simulink model "O_CloseLoop_Dynmodel"  (R2016b)
settings: Solver=VariableStepAuto  StartTime=0.0  StopTime=60.0  RelTol=1e-3
values from neighbouring files (symbols this model uses):
  MWS = JT9D_setup_everything_Dyn()    [BP_change_deter_data.m]    (also in JT9D_setup_everything_Dyn.m = input_set_0_0_100(MWS); make_train_data.m; sim_all_loss.m)
undefined symbols (not defined in the file or in its folder): Compressor, Lib_Turbo_Compressor_TMATS, stripchar_TMATS
libraries: Lib_Turbo_Duct_TMATS x5, Lib_Solve_DataOut_TMATS x5, Lib_Solve_OuterLoopIntegrator_TMATS x2, Lib_Turbo_Nozzle_TMATS x2, Lib_Turbo_Shaft_TMATS x2, Lib_Cntrl_FirstOrderActuator_TMATS x1, simulink x1, Lib_Cntrl_SimplePIcontroller_TMATS x1, Lib_Solve_IterNRSolverJC_TMATS x1, Lib_Turbo_Ambient_TMATS x1, Lib_Turbo_Burner_TMATS x1, Lib_Turbo_StaticCalc_TMATS x1
(part 1 of 2)
settings Model: Creator=zhang  LastModifiedBy=zhangshu
settings SolverCC: ZeroCrossAlgorithm=Adaptive

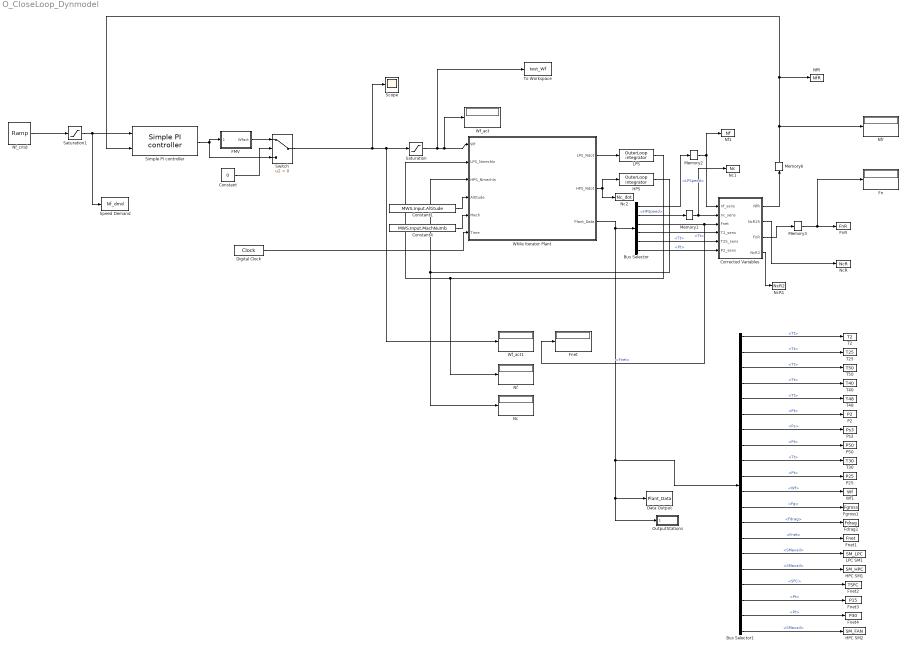
== system O_CloseLoop_Dynmodel ==
  Bus Selector : BusSelector  OutputSignals=Speed.LPSpeed,Speed.HPSpeed,Thrust.Fnet,StationData.S2.Tt,StationData.S24.Tt,StationData.S2.Pt
  Bus Selector1 : BusSelector  OutputSignals=StationData.S2.Tt,StationData.S24.Tt,StationData.S5.Tt,StationData.S4.Tt,StationData.S48.Tt,StationData.S2.Pt,StationData.S3.Ps,StationData.S5.Pt,StationData.S3.Tt,StationData.S24.Pt,Wf,Thrust.Fg,Data.Amb.Fdrag,Thrust.Fnet,Data.LPC.SMavail,Data.HPC.SMavail,SFC,StationData.S17.Pt,StationData.S3.Pt,Data.Fan.SMavail
  Constant : Constant  Value=0
  Constant1 : Constant  Value=MWS.Input.Altitude
  Constant4 : Constant  Value=MWS.Input.MachNumb
  Corrected Variables : Subsystem
  Data Output : ToWorkspace  VariableName=Plant_Data  SaveFormat=Timeseries  SampleTime=-1
  Digital Clock : DigitalClock  SampleTime=0.01
  FMV : Subsystem
  Fdrag1 : ToWorkspace  VariableName=Fdrag  SampleTime=-1
  Fgross1 : ToWorkspace  VariableName=Fgross  SampleTime=-1
  Fn : Display
  FnR : ToWorkspace  VariableName=FnR  SampleTime=-1
  Fnet : Display
  Fnet1 : ToWorkspace  VariableName=Fnet  SampleTime=-1
  Fnet2 : ToWorkspace  VariableName=TSFC  SampleTime=-1
  Fnet3 : ToWorkspace  VariableName=P15  SampleTime=-1
  Fnet4 : ToWorkspace  VariableName=P30  SampleTime=-1
  HPC SM1 : ToWorkspace  VariableName=SM_HPC  SampleTime=-1
  HPC SM2 : ToWorkspace  VariableName=SM_FAN  SampleTime=-1
  HPS : Lib_Solve_OuterLoopIntegrator_TMATS/OuterLoop integrator  OL_IC_M=MWS.Input.HP_Shaft
  LPC SM1 : ToWorkspace  VariableName=SM_LPC  SampleTime=-1
  LPS : Lib_Solve_OuterLoopIntegrator_TMATS/OuterLoop integrator  OL_IC_M=MWS.Input.LP_Shaft
  Memory{1..3,6} (4 alike) : Memory
  Nc : Display
  Nc1 : ToWorkspace  VariableName=Nc  SampleTime=-1
  Nc2 : ToWorkspace  VariableName=Nc_dot  SampleTime=-1
  NcR : ToWorkspace  VariableName=NcR  SampleTime=-1
  NcR1 : ToWorkspace  VariableName=NcR2  SampleTime=-1
  Nf : Display
  Nf1 : ToWorkspace  VariableName=Nf  SampleTime=-1
  NfR : ToWorkspace  VariableName=NfR  SampleTime=-1
  Nf_cmd : simulink/Sources/Ramp  slope=0  start=5  X0=3656.1
  Nfr : Display
  OutputStations : Subsystem
  P2 : ToWorkspace  VariableName=P2  SampleTime=-1
  P25 : ToWorkspace  VariableName=P25  SampleTime=-1
  P50 : ToWorkspace  VariableName=P50  SampleTime=-1
  Ps3 : ToWorkspace  VariableName=Ps3  SampleTime=-1
  Saturation : Saturate  UpperLimit=6  LowerLimit=0.2
  Saturation1 : Saturate  UpperLimit=3800  LowerLimit=1900
  Scope : Scope
  Simple PI controller : Lib_Cntrl_SimplePIcontroller_TMATS/Simple PI controller  Kp_M=0.0011  Ki_M=0.0556  PI_IC_M=MWS.Input.Wfin
  Speed Demand : ToWorkspace  VariableName=Nf_dmd  SaveFormat=Timeseries  SampleTime=-1
  Switch : Switch  Criteria=u2 > Threshold
  T2 : ToWorkspace  VariableName=T2  SampleTime=-1
  T25 : ToWorkspace  VariableName=T25  SampleTime=-1
  T30 : ToWorkspace  VariableName=T30  SampleTime=-1
  T40 : ToWorkspace  VariableName=T40  SampleTime=-1
  T48 : ToWorkspace  VariableName=T48  SampleTime=-1
  T50 : ToWorkspace  VariableName=T50  SampleTime=-1
  To Workspace : ToWorkspace  VariableName=test_Wf  SaveFormat=Timeseries  SampleTime=-1
  Wf1 : ToWorkspace  VariableName=Wf  SampleTime=-1
  Wf_act : Display
  Wf_act1 : Display
  While Iterator Plant : Subsystem  TreatAsAtomicUnit=on
  wires:
  Bus Selector/3 -> Fnet/1, Corrected Variables/3(Fnet)  "<Fnet>"
  Bus Selector/5 -> Corrected Variables/5(T25_sens)  "<Tt>"
  Bus Selector/6 -> Corrected Variables/6(P2_sens)  "<Pt>"
  While Iterator Plant/1(LPS_Ndot) -> LPS/1
  While Iterator Plant/2(HPS_Ndot) -> Nc2/1, HPS/1
  Constant4/1 -> While Iterator Plant/5(Mach)
  Constant1/1 -> While Iterator Plant/4(Altitude)
  Bus Selector1/11 -> Wf1/1  "<Wf>"
  Bus Selector1/3 -> T50/1  "<Tt>"
  Bus Selector1/2 -> T25/1  "<Tt>"
  Bus Selector1/1 -> T2/1  "<Tt>"
  Bus Selector1/4 -> T40/1  "<Tt>"
  Bus Selector1/5 -> T48/1  "<Tt>"
  Bus Selector1/6 -> P2/1  "<Pt>"
  Bus Selector1/7 -> Ps3/1  "<Ps>"
  Bus Selector1/8 -> P50/1  "<Pt>"
  Bus Selector1/9 -> T30/1  "<Tt>"
  Bus Selector1/10 -> P25/1  "<Pt>"
  Bus Selector1/15 -> LPC SM1/1  "<SMavail>"
  Bus Selector1/16 -> HPC SM1/1  "<SMavail>"
  HPS/1 -> Nc/1, While Iterator Plant/3(HPS_NmechIn)
  Corrected Variables/3(FnR) -> Memory3/1
  Memory1/1 -> Nc1/1, Corrected Variables/2(nc_sens)
  Memory2/1 -> Nf1/1, Corrected Variables/1(nf_sens)
  Corrected Variables/2(NcR25) -> NcR/1
  LPS/1 -> Nf/1, While Iterator Plant/2(LPS_NmechIn)
  Memory3/1 -> Fn/1, FnR/1
  Bus Selector/4 -> Corrected Variables/4(T2_sens)  "<Tt>"
  Bus Selector1/12 -> Fgross1/1  "<Fg>"
  Bus Selector1/14 -> Fnet1/1  "<Fnet>"
  Bus Selector1/13 -> Fdrag1/1  "<Fdrag>"
  Switch/1 -> Scope/1, Saturation/1, Wf_act1/1
  Bus Selector/1 -> Memory2/1  "<LPSpeed>"
  Bus Selector/2 -> Memory1/1  "<HPSpeed>"
  While Iterator Plant/3(Plant_Data) -> OutputStations/1(DataBus), Data Output/1, Bus Selector1/1, Bus Selector/1
  Saturation/1 -> To Workspace/1, While Iterator Plant/1(Wf), Wf_act/1
  Bus Selector1/17 -> Fnet2/1  "<SFC>"
  Digital Clock/1 -> While Iterator Plant/6(Time)
  Corrected Variables/1(NfR) -> Memory6/1
  Simple PI controller/1 -> FMV/1(Wfdmd), Switch/3
  FMV/1(Wfact) -> Switch/1
  Constant/1 -> Switch/2
  Memory6/1 -> Simple PI controller/2, NfR/1, Nfr/1
  Nf_cmd/1 -> Saturation1/1
  Corrected Variables/4(NcR2) -> NcR1/1
  Saturation1/1 -> Speed Demand/1, Simple PI controller/1
  Bus Selector1/18 -> Fnet3/1  "<Pt>"
  Bus Selector1/19 -> Fnet4/1  "<Pt>"
  Bus Selector1/20 -> HPC SM2/1  "<SMavail>"

== system O_CloseLoop_Dynmodel/Corrected Variables ==
  note: sqrt(theta)
  note: theta at
      | LPC outlet
  nf_sens : Inport
  nc_sens : Inport  Port=2
  Fnet : Inport  Port=3
  T2_sens : Inport  Port=4
  T25_sens : Inport  Port=5
  P2_sens : Inport  Port=6
  Divide{1..7} (7 alike) : Product  Inputs=*/
  Fn : Display
  Math Function : Math  Operator=sqrt  SaturateOnIntegerOverflow=on
  Math Function1 : Math  Operator=sqrt  SaturateOnIntegerOverflow=on
  nc_sens1 : InportShadow  Port=2
  std-day pressure (psi) : Constant  Value=MWS.C_PSTD
  std-day temp (degR) : Constant  Value=MWS.C_TSTD
  std-day temp (degR)1 : Constant  Value=MWS.C_TSTD
  NfR : Outport
  NcR25 : Outport  Port=2
  FnR : Outport  Port=3
  NcR2 : Outport  Port=4
  wires:
  Divide5/1 -> Divide6/2
  Fnet/1 -> Divide6/1
  Divide6/1 -> FnR/1
  std-day pressure (psi)/1 -> Divide5/2
  P2_sens/1 -> Divide5/1
  std-day temp (degR)/1 -> Divide3/2
  Divide1/1 -> Math Function/1
  T25_sens/1 -> Divide3/1
  std-day temp (degR)1/1 -> Divide1/2
  Divide2/1 -> NfR/1
  T2_sens/1 -> Divide1/1
  Divide3/1 -> Math Function1/1
  Math Function1/1 -> Divide4/2
  Divide4/1 -> NcR25/1
  nf_sens/1 -> Divide2/1
  Divide7/1 -> NcR2/1
  nc_sens/1 -> Divide4/1
  nc_sens1/1 -> Divide7/1
  Math Function/1 -> Fn/1, Divide7/2, Divide2/2

== system O_CloseLoop_Dynmodel/FMV ==
  Wfdmd : Inport
  1st order Actuator : Lib_Cntrl_FirstOrderActuator_TMATS/1st order Actuator  Gain_M=1  Tau_M=0.1  IC_M=MWS.Input.Wfin  MaxSat_M=5.0  MinSat_M=0  deadband_M=0.0  rateLimit_M=4.5
  Wf delay : TransportDelay  DelayTime=0.04  InitialOutput=MWS.Input.Wfin
  Wfact : Outport
  wires:
  Wf delay/1 -> Wfact/1  "Wfact"
  Wfdmd/1 -> 1st order Actuator/1
  1st order Actuator/1 -> Wf delay/1

== system O_CloseLoop_Dynmodel/OutputStations ==
  DataBus : Inport
  Bus Selector : BusSelector  OutputSignals=StationData.S1,StationData.S2,StationData.S21,StationData.S24,StationData.S3,StationData.S4,StationData.S45,StationData.S5,StationData.S7,StationData.S17,Data.Fan,Data.LPC,Data.HPC,Data.HPT,Data.LPT
  Data Output1 : ToWorkspace  VariableName=S1  SaveFormat=Timeseries  SampleTime=-1
  Data Output10 : ToWorkspace  VariableName=S17  SaveFormat=Timeseries  SampleTime=-1
  Data Output11 : ToWorkspace  VariableName=DFan  SaveFormat=Timeseries  SampleTime=-1
  Data Output12 : ToWorkspace  VariableName=DLPC  SaveFormat=Timeseries  SampleTime=-1
  Data Output13 : ToWorkspace  VariableName=DHPC  SaveFormat=Timeseries  SampleTime=-1
  Data Output14 : ToWorkspace  VariableName=DHPT  SaveFormat=Timeseries  SampleTime=-1
  Data Output15 : ToWorkspace  VariableName=DLPT  SaveFormat=Timeseries  SampleTime=-1
  Data Output2 : ToWorkspace  VariableName=S2  SaveFormat=Timeseries  SampleTime=-1
  Data Output3 : ToWorkspace  VariableName=S21  SaveFormat=Timeseries  SampleTime=-1
  Data Output4 : ToWorkspace  VariableName=S24  SaveFormat=Timeseries  SampleTime=-1
  Data Output5 : ToWorkspace  VariableName=S3  SaveFormat=Timeseries  SampleTime=-1
  Data Output6 : ToWorkspace  VariableName=S4  SaveFormat=Timeseries  SampleTime=-1
  Data Output7 : ToWorkspace  VariableName=S45  SaveFormat=Timeseries  SampleTime=-1
  Data Output8 : ToWorkspace  VariableName=S5  SaveFormat=Timeseries  SampleTime=-1
  Data Output9 : ToWorkspace  VariableName=S7  SaveFormat=Timeseries  SampleTime=-1
  wires:
  DataBus/1 -> Bus Selector/1
  Bus Selector/1 -> Data Output1/1  "<S1>"
  Bus Selector/2 -> Data Output2/1  "<S2>"
  Bus Selector/3 -> Data Output3/1  "<S21>"
  Bus Selector/4 -> Data Output4/1  "<S24>"
  Bus Selector/5 -> Data Output5/1  "<S3>"
  Bus Selector/6 -> Data Output6/1  "<S4>"
  Bus Selector/7 -> Data Output7/1  "<S45>"
  Bus Selector/8 -> Data Output8/1  "<S5>"
  Bus Selector/9 -> Data Output9/1  "<S7>"
  Bus Selector/10 -> Data Output10/1  "<S17>"
  Bus Selector/11 -> Data Output11/1  "<Fan>"
  Bus Selector/12 -> Data Output12/1  "<LPC>"
  Bus Selector/13 -> Data Output13/1  "<HPC>"
  Bus Selector/14 -> Data Output14/1  "<HPT>"
  Bus Selector/15 -> Data Output15/1  "<LPT>"

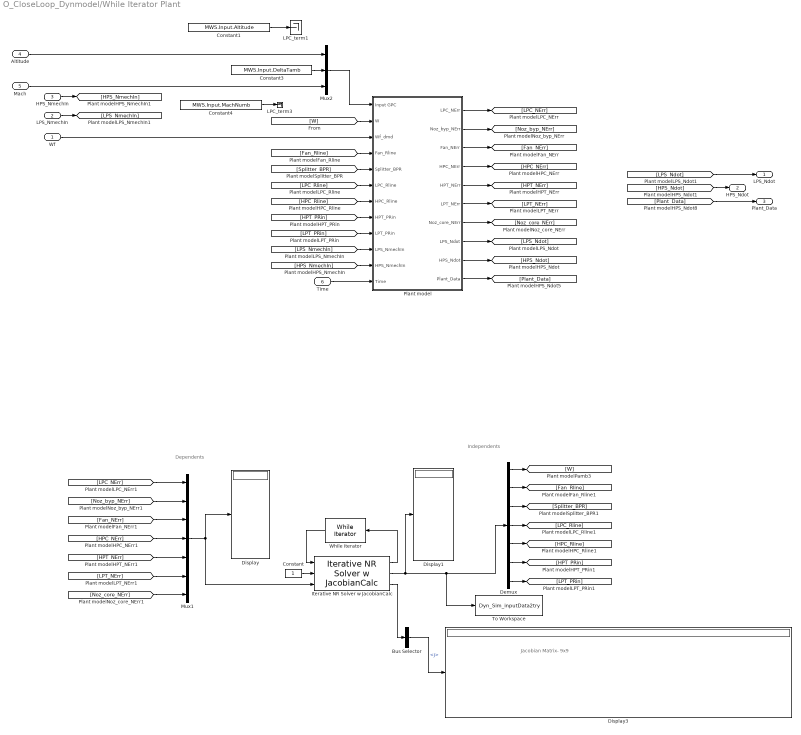
== system O_CloseLoop_Dynmodel/While Iterator Plant ==
  note: Jacobian Matrix- 9x9
  note: Dependents
  note: Independents
  Wf : Inport
  LPS_NmechIn : Inport  Port=2
  HPS_NmechIn : Inport  Port=3
  Altitude : Inport  Port=4
  Mach : Inport  Port=5
  Time : Inport  Port=6
  Bus Selector : BusSelector  OutputSignals=J
  Constant : Constant
  Constant1 : Constant  Value=MWS.Input.Altitude
  Constant3 : Constant  Value=MWS.Input.DeltaTamb
  Constant4 : Constant  Value=MWS.Input.MachNumb
  Demux : Demux  Outputs=7
  Display : Display
  Display1 : Display
  Display3 : Display
  Iterative NR Solver w JacobianCalc : Lib_Solve_IterNRSolverJC_TMATS/Iterative NR Solver w JacobianCalc  SJac_Per_M=[0.05 0.05 0.05 0.05 0.05 0.05 0.05]  SNR_IC_M=MWS.Input.NRICDyn  SNR_DX_M=5  SNR_Mx_M=100000  SNR_Mn_M=0.0001  SJacobianAttempts_M=20  Cond_Limits_M=0.0001
  LPC_term1 : Terminator
  LPC_term3 : Terminator
  Mux1 : Mux  Inputs=7
  Mux2 : Mux  Inputs=3
  Plant model : Subsystem
  To Workspace : ToWorkspace  VariableName=Dyn_Sim_inputData2try  SampleTime=-1
  While Iterator : WhileIterator  WhileBlockType=do-while  ShowIterationPort=on
  LPS_Ndot : Outport
  HPS_Ndot : Outport  Port=2
  Plant_Data : Outport  Port=3
  wires:
  Wf/1 -> Plant model/3(Wf_dmd)
  [Fan_Rline] -> Plant model/4(Fan_Rline)
  [Splitter_BPR] -> Plant model/5(Splitter_BPR)
  [LPC_Rline] -> Plant model/6(LPC_Rline)
  [HPC_Rline] -> Plant model/7(HPC_Rline)
  [HPT_PRin] -> Plant model/8(HPT_PRin)
  [LPT_PRin] -> Plant model/9(LPT_PRin)
  [LPS_NmechIn] -> Plant model/10(LPS_NmechIn)
  [HPS_NmechIn] -> Plant model/11(HPS_NmechIn)
  Plant model/1(LPC_NErr) -> [LPC_NErr]
  Plant model/2(Noz_byp_NErr) -> [Noz_byp_NErr]
  Plant model/3(Fan_NErr) -> [Fan_NErr]
  Plant model/4(HPC_NErr) -> [HPC_NErr]
  Plant model/5(HPT_NErr) -> [HPT_NErr]
  Plant model/6(LPT_NErr) -> [LPT_NErr]
  Plant model/7(Noz_core_NErr) -> [Noz_core_NErr]
  Plant model/8(LPS_Ndot) -> [LPS_Ndot]
  Plant model/9(HPS_Ndot) -> [HPS_Ndot]
  Demux/1 -> [W]
  Demux/7 -> [LPT_PRin]
  Demux/5 -> [HPC_Rline]
  Demux/6 -> [HPT_PRin]
  Demux/4 -> [LPC_Rline]
  Demux/2 -> [Fan_Rline]
  Demux/3 -> [Splitter_BPR]
  [Fan_NErr] -> Mux1/3
  [HPC_NErr] -> Mux1/4
  [Noz_byp_NErr] -> Mux1/2
  [HPT_NErr] -> Mux1/5
  [LPC_NErr] -> Mux1/1
  [LPT_NErr] -> Mux1/6
  [Noz_core_NErr] -> Mux1/7
  Iterative NR Solver w JacobianCalc/3 -> Bus Selector/1
  Mux1/1 -> Iterative NR Solver w JacobianCalc/3, Display/1
  Bus Selector/1 -> Display3/1  "<J>"
  Iterative NR Solver w JacobianCalc/2 -> To Workspace/1, Demux/1, Display1/1
  Iterative NR Solver w JacobianCalc/1 -> While Iterator/1
  HPS_NmechIn/1 -> [HPS_NmechIn]
  LPS_NmechIn/1 -> [LPS_NmechIn]
  [LPS_Ndot] -> LPS_Ndot/1
  [HPS_Ndot] -> HPS_Ndot/1
  Plant model/10(Plant_Data) -> [Plant_Data]
  [Plant_Data] -> Plant_Data/1
  Constant/1 -> Iterative NR Solver w JacobianCalc/2
  While Iterator/1 -> Iterative NR Solver w JacobianCalc/1
  [W] -> Plant model/2(W)
  Constant1/1 -> LPC_term1/1
  Constant3/1 -> Mux2/2
  Constant4/1 -> LPC_term3/1
  Mux2/1 -> Plant model/1(Input GPC)
  Mach/1 -> Mux2/3
  Altitude/1 -> Mux2/1
  Time/1 -> Plant model/12(Time)

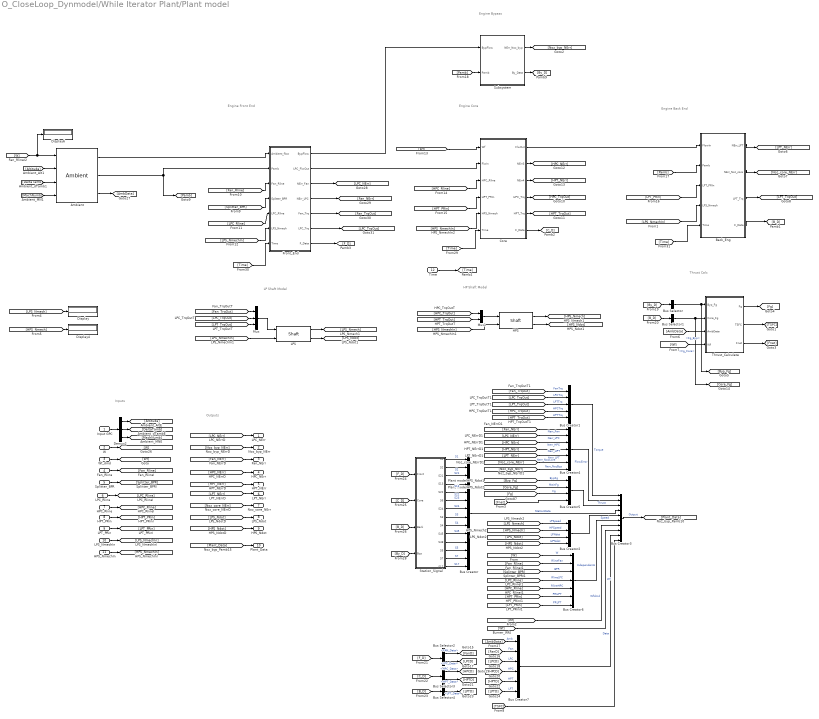
== system O_CloseLoop_Dynmodel/While Iterator Plant/Plant model ==
  note: LP Shaft Model
  note: Inputs
  note: Outputs
  note: Engine Core
  note: HP Shaft Model
  note: Engine Back End
  note: Engine Front End
  note: Thrust Calc
  note: Engine Bypass
  Input GPC : Inport
  W : Inport  Port=2
  Wf_dmd : Inport  Port=3
  Fan_Rline : Inport  Port=4
  Splitter_BPR : Inport  Port=5
  LPC_Rline : Inport  Port=6
  HPC_Rline : Inport  Port=7
  HPT_PRin : Inport  Port=8
  LPT_PRin : Inport  Port=9
  LPS_NmechIn : Inport  Port=10
  HPS_NmechIn : Inport  Port=11
  Time : Inport  Port=12
  Ambient : Lib_Turbo_Ambient_TMATS/Ambient  X_A_AltVec_M=5000*[-1 0 1 2 3 4 5 6 7 8 9 10 12 14 16]  T_A_TsVec_M=[536.51 518.67 500.84 483.03 465.22 447.41 429.62 411.84 394.06 389.97 389.97 389.97 389.97 392.25 397.69]  T_A_PsVec_M=[17.554 14.696 12.228 10.108 8.297 6.759 5.461 4.373 3.468 2.73 2.149 1.692 1.049 0.651 0.406]  AFARc_M=0  X_A_FARVec_M=[0; 0.0050; 0.0100; 0.0150; 0.0200; 0.0250; 0.0300]  T_A_RtArray_M="[0.0686;    0.0686;    0.0686;    0.0686;    0.0686;    0.0686;    0.0686]"  Y_A_TVec_M=[300 10000]  T_A_gammaArray_M=[ 1.4 1.4 1.4 1.4 1.4 1.4 1.4; 1.4 1.4 1.4 1.4 1.4 1.4 1.4]
  Back_Eng : Subsystem
  Bus Creator : BusCreator  Inputs=14
  Bus Creator1 : BusCreator  Inputs=5
  Bus Creator2 : BusCreator  Inputs=4
  Bus Creator3 : BusCreator  Inputs=10
  Bus Creator4 : BusCreator  Inputs=7
  Bus Creator5 : BusCreator  Inputs=4
  Bus Creator6 : BusCreator  Inputs=7
  Bus Creator7 : BusCreator  Inputs=6
  Bus Selector : BusSelector  OutputSignals=Fg_Byp
  Bus Selector1 : BusSelector  OutputSignals=Fg_Core
  Bus Selector2 : BusSelector  OutputSignals=FAN_Data,LPC_Data
  Bus Selector3 : BusSelector  OutputSignals=HPC_Data,HPT_Data
  Bus Selector4 : BusSelector  OutputSignals=LPT_Data
  Core : Subsystem
  Demux2 : Demux  Outputs=3
  Display : Display
  Display4 : Display
  Display6 : Display
  Front_End : Subsystem
  HPS : Lib_Turbo_Shaft_TMATS/Shaft  Shaft_Inertia_M=MWS.Shaft.Iner_hp
  LPS : Lib_Turbo_Shaft_TMATS/Shaft  Shaft_Inertia_M=MWS.Shaft.Iner_lp
  Mux : Mux  Inputs=3
  Mux1 : Mux  Inputs=2
  Station_Signal : Subsystem
  Subsystem : Subsystem
  Thrust_Calculate : Subsystem
  LPC_NErr : Outport
  Noz_byp_NErr : Outport  Port=2
  Fan_NErr : Outport  Port=3
  HPC_NErr : Outport  Port=4
  HPT_NErr : Outport  Port=5
  LPT_NErr : Outport  Port=6
  Noz_core_NErr : Outport  Port=7
  LPS_Ndot : Outport  Port=8
  HPS_Ndot : Outport  Port=9
  Plant_Data : Outport  Port=10
  wires:
  Fan_Rline/1 -> [Fan_Rline]
  HPS_NmechIn/1 -> [HPS_NmechIn]
  HPC_Rline/1 -> [HPC_Rline]
  LPT_PRin/1 -> [LPT_PRin]
  Wf_dmd/1 -> [Wf]
  Splitter_BPR/1 -> [Splitter_BPR]
  LPC_Rline/1 -> [LPC_Rline]
  HPT_PRin/1 -> [HPT_PRin]
  LPS_NmechIn/1 -> [LPS_NmechIn]
  Mux/1 -> LPS/1
  Mux1/1 -> HPS/1
  [LPT_TrqOut] -> Mux/3
  [Fan_TrqOut] -> Mux/1
  [HPT_TrqOut] -> Mux1/2
  [HPC_TrqOut] -> Mux1/1
  [LPC_TrqOut] -> Mux/2
  HPS/2 -> [HPS_Ndot]
  HPS/1 -> [HPS_Nmech]
  [HPS_NmechIn] -> HPS/2
  LPS/2 -> [LPS_Ndot]
  LPS/1 -> [LPS_Nmech]
  [LPS_NmechIn] -> LPS/2
  [LPC_NErr] -> LPC_NErr/1
  [Noz_byp_NErr] -> Noz_byp_NErr/1
  [Fan_NErr] -> Fan_NErr/1
  [HPC_NErr] -> HPC_NErr/1
  [HPT_NErr] -> HPT_NErr/1
  [LPT_NErr] -> LPT_NErr/1
  [Noz_core_NErr] -> Noz_core_NErr/1
  [LPS_Ndot] -> LPS_Ndot/1
  [HPS_Ndot] -> HPS_Ndot/1
  [Plant_Data] -> Plant_Data/1
  Station_Signal/6(S6) -> Bus Creator/6  "S23"
  Station_Signal/5(S22) -> Bus Creator/5  "S22"
  Station_Signal/7(S24) -> Bus Creator/7  "S24"
  Station_Signal/8(S3) -> Bus Creator/8  "S3"
  Station_Signal/4(S13) -> Bus Creator/4  "S13"
  Station_Signal/9(S4) -> Bus Creator/9  "S4"
  Station_Signal/3(S21) -> Bus Creator/3  "S21"
  Station_Signal/10(S45) -> Bus Creator/10  "S45"
  Station_Signal/2(S2) -> Bus Creator/2  "S2"
  Station_Signal/1(S1) -> Bus Creator/1  "S1"
  Station_Signal/12(S5) -> Bus Creator/12  "S5"
  Station_Signal/13(S7) -> Bus Creator/13  "S7"
  Station_Signal/14(S17) -> Bus Creator/14  "S17"
  Bus Creator/1 -> Bus Creator3/4  "StationData"
  Bus Creator2/1 -> Bus Creator3/5  "Speed"
  Bus Creator1/1 -> Bus Creator3/1  "Torque"
  Bus Creator3/1 -> [Plant_Data]  "Output"
  [Fan_NErr] -> Bus Creator4/1  "Nerr_Fan"
  [Noz_byp_NErr] -> Bus Creator4/7  "Nerr_NozByp"
  [LPC_NErr] -> Bus Creator4/2  "Nerr_LPC"
  [HPC_NErr] -> Bus Creator4/3  "Nerr_HPC"
  [HPT_NErr] -> Bus Creator4/4  "Nerr_HPT"
  [LPT_NErr] -> Bus Creator4/5  "Nerr_LPT"
  [Noz_core_NErr] -> Bus Creator4/6  "Nerr_NozCore"
  [Fan_TrqOut] -> Bus Creator1/1  "FanTrq"
  [LPC_TrqOut] -> Bus Creator1/2  "LPCTrq"
  [HPC_TrqOut] -> Bus Creator1/4  "HPCTrq"
  [HPT_TrqOut] -> Bus Creator1/5  "HPTTrq"
  [LPT_TrqOut] -> Bus Creator1/3  "LPTTrq"
  [Byp_Fg] -> Bus Creator5/1  "BypFg"
  [Core_Fg] -> Bus Creator5/2  "MainFg"
  [Fg] -> Bus Creator5/3  "Fg"
  [LPS_Nmech] -> Bus Creator2/1  "LPSpeed"
  [HPS_Nmech] -> Bus Creator2/2  "HPSpeed"
  [LPS_Ndot] -> Bus Creator2/3  "LPNdot"
  [HPS_Ndot] -> Bus Creator2/4  "HPNdot"
  [HPT_PRin] -> Bus Creator6/6  "PRHPT"
  [HPC_Rline] -> Bus Creator6/5  "RlineHPC"
  [Fan_Rline] -> Bus Creator6/2  "RlineFan"
  [Splitter_BPR] -> Bus Creator6/3  "BPR"
  [LPC_Rline] -> Bus Creator6/4  "RlineLPC"
  [LPT_PRin] -> Bus Creator6/7  "PRLPT"
  Bus Creator4/1 -> Bus Creator3/2  "FlowError"
  Bus Creator5/1 -> Bus Creator3/3  "Thrust"
  Bus Creator6/1 -> Bus Creator3/6  "Independents"
  [Wf] -> Bus Creator3/7  "Wfdmd"
  [Wf] -> Bus Creator3/8  "Wf"
  [LPCD] -> Bus Creator7/3  "LPC"
  [FanD] -> Bus Creator7/2  "Fan"
  [HPCD] -> Bus Creator7/4  "HPC"
  [HPTD] -> Bus Creator7/5  "HPT"
  [LPTD] -> Bus Creator7/6  "LPT"
  Bus Creator7/1 -> Bus Creator3/9  "Data"
  [W] -> Display6/1, Ambient/1
  [Altitude] -> Ambient/2
  [DeltaTamb] -> Ambient/3
  [MachNumb] -> Ambient/4
  Ambient/3 -> [AmbData]
  Input GPC/1 -> Demux2/1
  Demux2/1 -> [Altitude]
  Demux2/2 -> [DeltaTamb]
  Demux2/3 -> [MachNumb]
  W/1 -> [W]
  [W] -> Bus Creator6/1  "W"
  [Fnet] -> Bus Creator5/4
  [TSFC] -> Bus Creator3/10
  Ambient/1 -> Front_End/1(Ambient_flow)
  Ambient/2 -> Front_End/2(Pamb), [Pamb]
  [Splitter_BPR] -> Front_End/4(Splitter_BPR)
  [Fan_Rline] -> Front_End/3(Fan_Rline)
  [LPC_Rline] -> Front_End/5(LPC_Rline)
  [LPS_NmechIn] -> Front_End/6(LPS_Nmech)
  Front_End/3(NErr_Fan) -> [LPC_NErr]
  Front_End/4(NErr_LPC) -> [Fan_NErr]
  Front_End/5(Fan_Trq) -> [Fan_TrqOut]
  Front_End/6(LPC_Trq) -> [LPC_TrqOut]
  Front_End/1(BypFlow) -> Subsystem/1(BypFlow)
  Front_End/2(LPC_FlwOut) -> Core/2(FlwIn)
  [Wf] -> Core/1(Wf)
  [HPC_Rline] -> Core/3(HPC_Rline)
  [HPT_PRin] -> Core/4(HPT_PRIn)
  [HPS_NmechIn] -> Core/5(HPS_Nmech)
  Core/4(HPC_Trq) -> [HPC_TrqOut]
  Core/5(HPT_Trq) -> [HPT_TrqOut]
  Core/2(NErr3) -> [HPC_NErr]
  Core/3(NErr4) -> [HPT_NErr]
  Core/1(FlwOut) -> Back_Eng/1(FlowIn)
  [LPS_NmechIn] -> Back_Eng/4(LPS_Nmech)
  [LPT_PRin] -> Back_Eng/3(LPT_PRIn)
  Back_Eng/1(NErr_LPT) -> [LPT_NErr]
  Back_Eng/2(NErr_Noz_core) -> [Noz_core_NErr]
  Back_Eng/3(LPT_Trq) -> [LPT_TrqOut]
  [Pamb] -> Back_Eng/2(Pamb)
  [Pamb] -> Subsystem/2(Pamb)
  Subsystem/1(NErr_Noz_byp) -> [Noz_byp_NErr]
  [LPS_Nmech] -> Display/1
  [HPS_Nmech] -> Display4/1
  [AmbData] -> Thrust_Calculate/3(AmbData)
  [Wf] -> Thrust_Calculate/4(Wf)
  Thrust_Calculate/2(TSFC) -> [TSFC]
  Subsystem/2(By_Data) -> [By_D]
  Back_Eng/4(C_Data) -> [B_D]
  Core/6(C_Data) -> [C_D]
  Front_End/7(F_Data) -> [F_D]
  [By_D] -> Bus Selector/1
  Bus Selector/1 -> [Byp_Fg], Thrust_Calculate/1(Byp_Fg)  "<Fg_Byp>"
  [B_D] -> Bus Selector1/1
  Bus Selector1/1 -> [Core_Fg], Thrust_Calculate/2(Core_Fg)  "<Fg_Core>"
  [F_D] -> Bus Selector2/1
  Bus Selector2/1 -> [FanD]  "<FAN_Data>"
  Bus Selector2/2 -> [LPCD]  "<LPC_Data>"
  [C_D] -> Bus Selector3/1
  Bus Selector3/1 -> [HPCD]  "<HPC_Data>"
  Bus Selector3/2 -> [HPTD]  "<HPT_Data>"
  [B_D] -> Bus Selector4/1
  Bus Selector4/1 -> [LPTD]  "<LPT_Data>"
  Station_Signal/11(S48) -> Bus Creator/11
  [F_D] -> Station_Signal/1(Front)
  [C_D] -> Station_Signal/2(Core)
  [B_D] -> Station_Signal/3(Back)
  [By_D] -> Station_Signal/4(Byp)
  Thrust_Calculate/1(Fg) -> [Fg]
  Thrust_Calculate/3(Fnet) -> [Fnet]
  [AmbData] -> Bus Creator7/1  "Amb"
  Time/1 -> [Time]
  [Time] -> Core/6(Time)
  [Time] -> Front_End/7(Time)
  [Time] -> Back_Eng/5(Time)

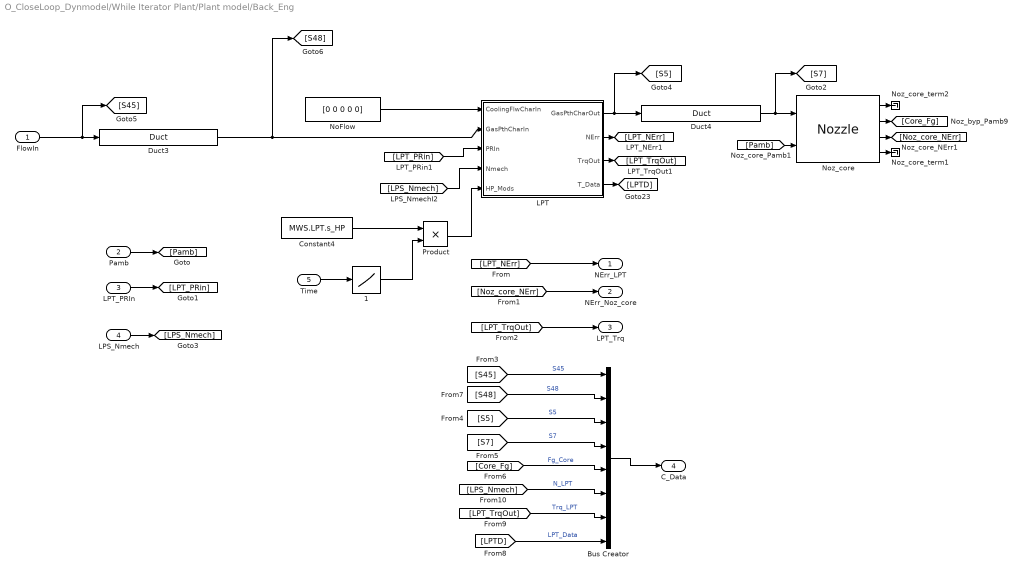
== system O_CloseLoop_Dynmodel/While Iterator Plant/Plant model/Back_Eng ==
  FlowIn : Inport
  Pamb : Inport  Port=2
  LPT_PRIn : Inport  Port=3
  LPS_Nmech : Inport  Port=4
  Time : Inport  Port=5
  1 : Lookup  InputValues=MWS.HP_in.t  Table=MWS.HP_in.scaled
  Bus Creator : BusCreator  Inputs=8
  Constant4 : Constant  Value=MWS.LPT.s_HP
  Duct3 : Lib_Turbo_Duct_TMATS/Duct  dP_M=MWS.Duct.dP3
  Duct4 : Lib_Turbo_Duct_TMATS/Duct  dP_M=MWS.Duct.dP4
  LPT : Subsystem  mask(T-MATS: Turbine, NPSS Library Block){X_T_Map_PRVec_M=MWS.LPT.PRVec, Y_T_Map_NcVec_M=MWS.LPT.NcVec, T_T_Map_WcArray_M=MWS.LPT.WcArray, T_T_Map_EffArray_M=MWS.LPT.EffArray, s_T_Nc_M=MWS.LPT.s_Nc, s_T_Wc_M=MWS.LPT.s_Wc, s_T_PR_M=MWS.LPT.s_PR, s_T_Eff_M=MWS.LPT.s_eff, ConfigNPSS_M=1, Scale_M=none, CFlwEn_M=off, T_CoolFlwPos_M=0, iDesign_M=MWS.iDes, NcDes_M=105.038, EffDes_M=.9323, PRDes_M=6.420, NDes_M=3667.6, FVar_M=strcat('iDes_',stripchar_TMATS(gcb),'.bin'), BlkNm_M=double(gcb), HP_M=on}
      mask prompts: X_T_Map_PRVec_M "X_T_Map_PRVec_M - Turbine Map Pressure Ratio Vector (X-axis)(nx1)"; Y_T_Map_NcVec_M "Y_T_Map_NcVec_M - Turbine Map Corrected Speed Vector (Y-axis)(mx1)"; T_T_Map_WcArray_M "T_T_Map_WcArray_M - Turbine Map Flow Array (Wc=f(Nc,PR))(mxn)"; T_T_Map_EffArray_M "T_T_Map_EffArray_M - Turbine Map Efficiency Array (Eff = f(Nc,PR))(mxn)"; s_T_Nc_M "s_T_Nc_M - Corrected Speed Scalar Constant (T_Nc)"; s_T_Wc_M "s_T_Wc_M - Flow Scalar Constant (T_Wc)"; s_T_PR_M "s_T_PR_M - Pressure Ratio Scalar Constant (T_PR)"; s_T_Eff_M "s_T_Eff_M - Efficiency Scalar Constant (T_Eff)"; ConfigNPSS_M "ConfigNPSS_M - configure for type usage of maps and constants"; Scale_M "Scalars"; CFlwEn_M "CFlwEn_M - Cooling Flow Enable [0-off, 1-on]"; T_CoolFlwPos_M "T_CoolFlwPos_M - Cooling Flow position [0 at inlet,  1 at exit] (cx1)"; iDesign_M "iDesign_M - Design fork (0 - Enable iDes, 1 - Use iDes Scalars, 2 - Use Specified Input Scalars)"; NcDes_M "NcDes_M - map Design Corrected Shaft Speed [rpm]"; EffDes_M "EffDes_M - Design Efficiency [frac]"; PRDes_M "PRDes_M - map Design Pressure Ratio [frac]"; NDes_M "NDes_M - Design Shaft Speed [rpm]"; FVar_M "FVar_M - File name for iDes Variables"; BlkNm_M "Block name as double for Simulink output"; HP_M "HP_M - Enable Health Parameter input (2x1 vector)"
      mask help: This block simulates the performance of a turbine using basic thermodynamic equations, properties, and table lookups. This block has been updated to be more similar to the baseline NPSS turbine module. Updates include removing the standard day components of the Nc and Wc calculations and updating the Flow error term to use input flow only, which translates to a turbine map in which Wc is defined as input flow only.
      mask init:
      | if iDesign_M == 1
      |     P = load(FVar_M);
      |     s_T_Nc_M = P(1);
      |     s_T_Wc_M = P(2);
      |     s_T_PR_M = P(3);
      |     s_T_Eff_M = P(4);
      | end
      | 
      | if length(X_T_Map_PRVec_M) ~= size(T_T_Map_WcArray_M,2)
      |     warning('number of columns in T_T_Map_WcArray_M does not match length of X_T_Map_PRVec_M');
      | end
      | if length(X_T_Map_PRVec_M) ~= size(T_T_Map_EffArray_M,2)
      |     warning('number of columns in T_T_Map_EffArray_M does not match length of X_T_Map_PRVec_M');
      | end
      | if length(Y_T_Map_NcVec_M) ~= size(T_T_Map_WcArray_M,1)
      |     warning('number of rows in T_T_Map_WcArray_M does not match length of Y_T_Map_NcVec_M');
      | end
      | if length(Y_T_Map_NcVec_M) ~= size(T_T_Map_EffArray_M,1)
      |     warning('number of rows in T_T_Map_EffArray_M does not match length of Y_T_Map_NcVec_M');
      | end
      | 
      | % produce warning if Health Parameters are enabled and IDesign is set to 0
      | if HP_M && iDesign_M == 0
      |     warning('iDesign is set to 0 (model on design) and health parameters are enabled. HP values will be ignored.');
      | end
      | 
      | %Manage Health Parameter inputs
      | if HP_M == 1
      |     if strcmp(get_param([BlkNm_M '/HP_Mods'],'BlockType'),'Constant')
      |         MSK_ReplaceBlock_TMATS([BlkNm_M '/HP_Mods'],'built-in/Inport');
      |     end
      |     set_param([BlkNm_M '/HP_Mods'],'Port',num2str(5));
      | elseif HP_M == 0
      |     if strcmp(get_param([BlkNm_M '/HP_Mods'],'BlockType'),'Inport')
      |         MSK_ReplaceBlock_TMATS([BlkNm_M '/HP_Mods'],'built-in/Constant');
      |         set_param([BlkNm_M '/HP_Mods'],'Value','[0, 0]');
      |     end
      | end
      mask Help: web(which('Turbo_TMATS_TrbNPSS.html'),'-helpbrowser')
      mask TypeOptions Scale_M: none | user defined | iDesign
      mask Callback CFlwEn_M: MSK_SEC_Enables_TMATS('CFlwEn_M',12,'en')
      mask Callback iDesign_M:
      | MSK_SEC_Enables_Ides_TMATS('iDesign_M',[5 6 7 8],'G1')
      | MSK_SEC_Enables_Ides_TMATS('iDesign_M',[14 15 16 17],'G2')
      | MSK_SEC_Enables_Ides_TMATS('iDesign_M',[18],'G3')
      mask DialogControl Control2 Prompt: Plot Map
      mask DialogControl Control2 Callback: MSK_PlotTMap_TMATS()
  NoFlow : Constant  Value=[0 0 0 0 0]
  Noz_core : Lib_Turbo_Nozzle_TMATS/Nozzle  SWType_M=Convergent  N_TArea_M=MWS.Noz.Ath  N_EArea_M=110.7  N_FL_M=0.00  X_N_TtVec2_M=[300 2000]  T_N_TGArray_M=[1 1]  X_N_PEQPaVec_M=[0 10000]  T_N_CdThArray_M=[1 1]  T_N_CvArray_M=MWS.Noz.CvArray  CfgEn_M=off  T_N_CfgArray_M=[1 1]  X_N_FARVec_M=[0; 0.0050; 0.0100; 0.0150; 0.0200; 0.0250; 0.0300]  T_N_RtArray_M="[0.0686;    0.0686;    0.0686;    0.0686;    0.0686;    0.0686;    0.0686]"  Y_N_TtVec_M=[300 2000]  T_N_MAP_gammaArray_M=[ 1.4 1.4 1.4 1.4 1.4 1.4 1.4; 1.4 1.4 1.4 1.4 1.4 1.4 1.4]  iDesign_M=MWS.iDes  WDes_M=113.51  FVar_M=strcat('iDes_',stripchar_TMATS(gcb),'.bin')
  Noz_core_term1 : Terminator
  Noz_core_term2 : Terminator
  Product : Product
  NErr_LPT : Outport
  NErr_Noz_core : Outport  Port=2
  LPT_Trq : Outport  Port=3
  C_Data : Outport  Port=4
  wires:
  [S7] -> Bus Creator/4  "S7"
  [S48] -> Bus Creator/2  "S48"
  [Core_Fg] -> Bus Creator/5  "Fg_Core"
  [S5] -> Bus Creator/3  "S5"
  Bus Creator/1 -> C_Data/1
  [LPS_Nmech] -> Bus Creator/6  "N_LPT"
  [LPT_TrqOut] -> Bus Creator/7  "Trq_LPT"
  [LPTD] -> Bus Creator/8  "LPT_Data"
  Pamb/1 -> [Pamb]
  FlowIn/1 -> [S45], Duct3/1
  Duct4/1 -> [S7], Noz_core/1
  [Pamb] -> Noz_core/2
  Noz_core/3 -> [Noz_core_NErr]
  Noz_core/4 -> Noz_core_term1/1
  LPT/1(GasPthCharOut) -> [S5], Duct4/1
  LPT/4(T_Data) -> [LPTD]
  LPT/2(NErr) -> [LPT_NErr]
  [LPS_Nmech] -> LPT/4(Nmech)
  NoFlow/1 -> LPT/1(CoolingFlwCharIn)
  LPT/3(TrqOut) -> [LPT_TrqOut]
  Noz_core/2 -> [Core_Fg]
  [LPT_PRin] -> LPT/3(PRIn)
  Noz_core/1 -> Noz_core_term2/1
  [Noz_core_NErr] -> NErr_Noz_core/1
  [S45] -> Bus Creator/1  "S45"
  [LPT_NErr] -> NErr_LPT/1
  [LPT_TrqOut] -> LPT_Trq/1
  LPS_Nmech/1 -> [LPS_Nmech]
  LPT_PRIn/1 -> [LPT_PRin]
  Duct3/1 -> LPT/2(GasPthCharIn), [S48]
  Constant4/1 -> Product/1
  Product/1 -> LPT/5(HP_Mods)
  1/1 -> Product/2
  Time/1 -> 1/1

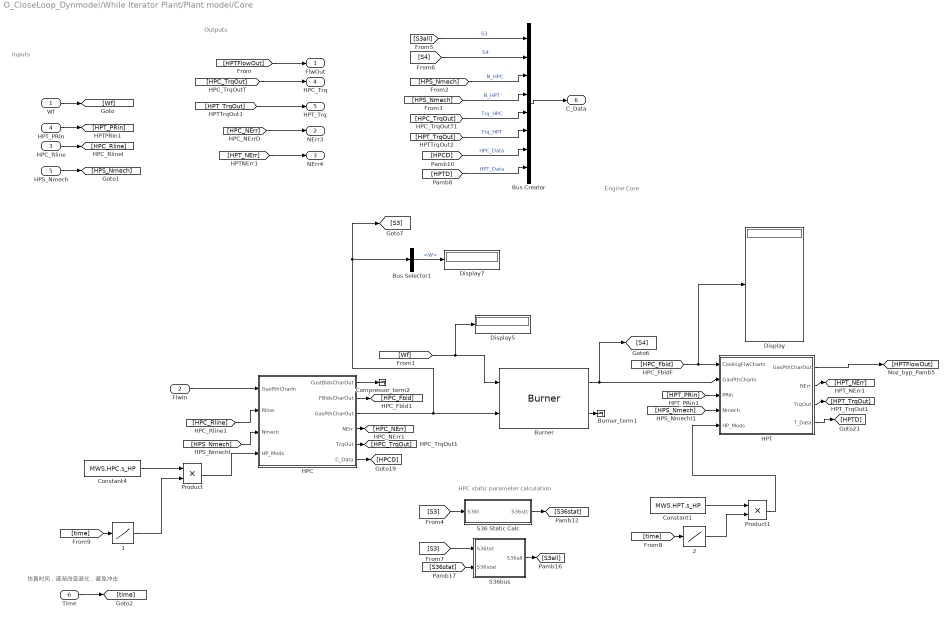
== system O_CloseLoop_Dynmodel/While Iterator Plant/Plant model/Core ==
  note: Engine Core
  note: Inputs
  note: Outputs
  note: HPC static parameter calculation
  note: 仿真时间，逐渐改变退化，避免冲击
  Wf : Inport
  FlwIn : Inport  Port=2
  HPC_Rline : Inport  Port=3
  HPT_PRIn : Inport  Port=4
  HPS_Nmech : Inport  Port=5
  Time : Inport  Port=6
  1 : Lookup  InputValues=MWS.HP_in.t  Table=MWS.HP_in.scaled
  2 : Lookup  InputValues=MWS.HP_in.t  Table=MWS.HP_in.scaled
  Burner : Lib_Turbo_Burner_TMATS/Burner  LHVEn_M=on  LHV_M=18400  Eff_M=0.994  hFuel_M=-1200  dPnormBurner_M=MWS.Burn.dP
  Burner_term1 : Terminator
  Bus Creator : BusCreator  Inputs=8
  Bus Selector1 : BusSelector  OutputSignals=W
  Compressor_term2 : Terminator
  Constant1 : Constant  Value=MWS.HPT.s_HP
  Constant4 : Constant  Value=MWS.HPC.s_HP
  Display : Display
  Display5 : Display
  Display7 : Display
  HPC : Subsystem  mask(T-MATS: Compressor Library Block){X_C_RlineVec_M=MWS.HPC.RlineVec, Z_C_AlphaVec_M=1, Y_C_Map_NcVec_M=MWS.HPC.NcVec, T_C_Map_WcArray_M=MWS.HPC.WcArray, T_C_Map_PRArray_M=MWS.HPC.PRArray, T_C_Map_EffArray_M=MWS.HPC.EffArray, s_C_Nc_M=MWS.HPC.s_Nc, s_C_Wc_M=MWS.HPC.s_Wc, s_C_PR_M=MWS.HPC.s_PR, s_C_Eff_M=MWS.HPC.s_eff, SL_M=off, Scale_M=iDesign, CBLDEN_M=off, C_CBD_M=0, C_CBFht_M=0.5, C_CBFPt_M=0.5, FBLDEN_M=on, C_FBD_M=MWS.HPC.Fbld, C_BFht_M=MWS.HPC.Fblde, C_BFPt_M=MWS.HPC.Fbldp, DefSMEn_M=off, SRline_M=1, X_C_Map_WcSurgeVec_M=[164.18 183.5 202.63 209.9986], T_C_Map_PRSurgeVec_M=[19.61 23.26 26.69 27.6439], iDesign_M=MWS.iDes, NcDes_M=0.995, EffDes_M=.8651, PRDes_M=5.609, RlineDes_M=2.0424, FVar_M=strcat('iDes_',stripchar_TMATS(gcb),'.bin'), BlkNm_M=double(gcb), HP_M=on}
      mask prompts: X_C_RlineVec_M "X_C_RlineVec_M - Compressor Map Rline Vector (X-axis)(nx1)"; Z_C_AlphaVec_M "Z_C_Map_AlphaVec_M - Compressor Alpha Vector (Z-axis)(rx1)"; Y_C_Map_NcVec_M "Y_C_Map_NcVec_M - Compressor Map Corrected Speed Vector (Y-axis)(mx1)"; T_C_Map_WcArray_M "T_C_Map_WcArray_M - Compressor Map Flow Array (Wc = f(Nc, Rline))(mxn)"; T_C_Map_PRArray_M "T_C_Map_PRArray_M - Compressor Map Pressure Ratio Array (PR = f(Nc, Rline))(mxn)"; T_C_Map_EffArray_M "T_C_Map_EffArray_M - Compressor Map Efficiency Array (Eff = f(Nc, Rline)(mxn)"; s_C_Nc_M "s_C_Nc_M - Corrected Speed Scalar Constant (C_Nc)"; s_C_Wc_M "s_C_Wc_M - Flow Scalar Constant (C_Wc)"; s_C_PR_M "s_C_PR_M - Pressure Ratio Scalar Constant (C_PR)"; s_C_Eff_M "s_C_Eff_M - Efficiency Scalar Constant (C_Eff)"; SL_M "Include surge line"; Scale_M "Scalars"; CBLDEN_M "CBLDEN_M - Customer Bleed Enable [0 - off, 1 - on]"; C_CBD_M "C_CBD_M - Customer or Flow based Bleed Demand[pps] (cbx1)"; C_CBFht_M "C_CBFht_M - Customer or Flow based Bleed Fractional enthalpy[frac] (cbx1)"; C_CBFPt_M "C_CBFPt_M - Customer or Flow based Bleed Fractional Total Pressure[frac] (cbx1)"; FBLDEN_M "FBLDEN_M - Fractional Bleed Enable [0 - off, 1 - on]"; C_FBD_M "C_FBD_M - Fractional Bleed Demand[frac] (bx1)"; C_BFht_M "C_BFht_M - Engine Bleed Fractional Enthalpy[frac] (bx1)"; C_BFPt_M "C_BFPt_M - Engine Bleed Fractional Total Pressure[frac] (bx1)"; DefSMEn_M "DefSMEn_M - Use map default (Rline = 1) surge line"; SRline_M "SRline_M - Rline defined as surge line"; X_C_Map_WcSurgeVec_M "X_C_Map_WcSurgeVec_M - map Compensated flow surge vector (sx1)"; T_C_Map_PRSurgeVec_M "T_C_Map_PRSurgeVec_M - map Surge Line Pressure Ratio vector (sx1)"; iDesign_M "iDesign_M - Design fork (0 - Enable iDes, 1 - Use iDes Scalars, 2 - Use Specified Input Scalars)"; NcDes_M "NcDes_M - map Design Corrected Shaft Speed [rpm]"; EffDes_M "EffDes_M  - Design Efficiency [frac]"; PRDes_M "PRDes_M - Design Pressure Ratio [frac]"; RlineDes_M "RlineDes_M - map Design Rline"; FVar_M "FVar_M - File name for iDes Variables"; BlkNm_M "Block name as double for Simulink output"; HP_M "HP_M - Enable Health Parameter input (3x1 vector)"
      mask help: This block simulates the performance of a compressor using basic thermodynamic equations, properties, and table lookups.
      mask init:
      | MSK_CompInit_TMATS
      mask Help: web(which('Turbo_TMATS_Cmp.html'),'-helpbrowser')
      mask TypeOptions Scale_M: none | user defined | iDesign
      mask Callback CBLDEN_M: MSK_SEC_Enables_TMATS('CBLDEN_M',[14 15 16],'en')
      mask Callback FBLDEN_M: MSK_SEC_Enables_TMATS('FBLDEN_M',[18 19 20],'en')
      mask Callback DefSMEn_M:
      | MSK_SEC_Enables_TMATS('DefSMEn_M',[23 24],'dis')
      | MSK_SEC_Enables_TMATS('DefSMEn_M',[22],'en')
      mask Callback iDesign_M:
      | MSK_SEC_Enables_Ides_TMATS('iDesign_M',[7 8 9 10],'G1')
      | MSK_SEC_Enables_Ides_TMATS('iDesign_M',[26 27 28 29],'G2')
      | MSK_SEC_Enables_Ides_TMATS('iDesign_M',[30],'G3')
      mask DialogControl Control2 Prompt: Plot Map
      mask DialogControl Control2 Callback: MSK_PlotCMap_TMATS()
  HPT : Subsystem  mask(T-MATS: Turbine, NPSS Library Block){X_T_Map_PRVec_M=MWS.HPT.PRVec, Y_T_Map_NcVec_M=MWS.HPT.NcVec, T_T_Map_WcArray_M=MWS.HPT.WcArray, T_T_Map_EffArray_M=MWS.HPT.EffArray, s_T_Nc_M=MWS.HPT.s_Nc, s_T_Wc_M=MWS.HPT.s_Wc, s_T_PR_M=MWS.HPT.s_PR, s_T_Eff_M=MWS.HPT.s_eff, ConfigNPSS_M=1, Scale_M=none, CFlwEn_M=on, T_CoolFlwPos_M=MWS.HPT.Cool, iDesign_M=MWS.iDes, NcDes_M=99.031, EffDes_M=.9133, PRDes_M=4.930, NDes_M=7390, FVar_M=strcat('iDes_',stripchar_TMATS(gcb),'.bin'), BlkNm_M=double(gcb), HP_M=on}
      mask prompts: X_T_Map_PRVec_M "X_T_Map_PRVec_M - Turbine Map Pressure Ratio Vector (X-axis)(nx1)"; Y_T_Map_NcVec_M "Y_T_Map_NcVec_M - Turbine Map Corrected Speed Vector (Y-axis)(mx1)"; T_T_Map_WcArray_M "T_T_Map_WcArray_M - Turbine Map Flow Array (Wc=f(Nc,PR))(mxn)"; T_T_Map_EffArray_M "T_T_Map_EffArray_M - Turbine Map Efficiency Array (Eff = f(Nc,PR))(mxn)"; s_T_Nc_M "s_T_Nc_M - Corrected Speed Scalar Constant (T_Nc)"; s_T_Wc_M "s_T_Wc_M - Flow Scalar Constant (T_Wc)"; s_T_PR_M "s_T_PR_M - Pressure Ratio Scalar Constant (T_PR)"; s_T_Eff_M "s_T_Eff_M - Efficiency Scalar Constant (T_Eff)"; ConfigNPSS_M "ConfigNPSS_M - configure for type usage of maps and constants"; Scale_M "Scalars"; CFlwEn_M "CFlwEn_M - Cooling Flow Enable [0-off, 1-on]"; T_CoolFlwPos_M "T_CoolFlwPos_M - Cooling Flow position [0 at inlet,  1 at exit] (cx1)"; iDesign_M "iDesign_M - Design fork (0 - Enable iDes, 1 - Use iDes Scalars, 2 - Use Specified Input Scalars)"; NcDes_M "NcDes_M - map Design Corrected Shaft Speed [rpm]"; EffDes_M "EffDes_M - Design Efficiency [frac]"; PRDes_M "PRDes_M - map Design Pressure Ratio [frac]"; NDes_M "NDes_M - Design Shaft Speed [rpm]"; FVar_M "FVar_M - File name for iDes Variables"; BlkNm_M "Block name as double for Simulink output"; HP_M "HP_M - Enable Health Parameter input (2x1 vector)"
      mask help: This block simulates the performance of a turbine using basic thermodynamic equations, properties, and table lookups. This block has been updated to be more similar to the baseline NPSS turbine module. Updates include removing the standard day components of the Nc and Wc calculations and updating the Flow error term to use input flow only, which translates to a turbine map in which Wc is defined as input flow only.
      mask init:
      | if iDesign_M == 1
      |     P = load(FVar_M);
      |     s_T_Nc_M = P(1);
      |     s_T_Wc_M = P(2);
      |     s_T_PR_M = P(3);
      |     s_T_Eff_M = P(4);
      | end
      | 
      | if length(X_T_Map_PRVec_M) ~= size(T_T_Map_WcArray_M,2)
      |     warning('number of columns in T_T_Map_WcArray_M does not match length of X_T_Map_PRVec_M');
      | end
      | if length(X_T_Map_PRVec_M) ~= size(T_T_Map_EffArray_M,2)
      |     warning('number of columns in T_T_Map_EffArray_M does not match length of X_T_Map_PRVec_M');
      | end
      | if length(Y_T_Map_NcVec_M) ~= size(T_T_Map_WcArray_M,1)
      |     warning('number of rows in T_T_Map_WcArray_M does not match length of Y_T_Map_NcVec_M');
      | end
      | if length(Y_T_Map_NcVec_M) ~= size(T_T_Map_EffArray_M,1)
      |     warning('number of rows in T_T_Map_EffArray_M does not match length of Y_T_Map_NcVec_M');
      | end
      | 
      | % produce warning if Health Parameters are enabled and IDesign is set to 0
      | if HP_M && iDesign_M == 0
      |     warning('iDesign is set to 0 (model on design) and health parameters are enabled. HP values will be ignored.');
      | end
      | 
      | %Manage Health Parameter inputs
      mask Help: web(which('Turbo_TMATS_TrbNPSS.html'),'-helpbrowser')
      mask TypeOptions Scale_M: none | user defined | iDesign
      mask Callback CFlwEn_M: MSK_SEC_Enables_TMATS('CFlwEn_M',12,'en')
      mask Callback iDesign_M:
      | MSK_SEC_Enables_Ides_TMATS('iDesign_M',[5 6 7 8],'G1')
      | MSK_SEC_Enables_Ides_TMATS('iDesign_M',[14 15 16 17],'G2')
      | MSK_SEC_Enables_Ides_TMATS('iDesign_M',[18],'G3')
      mask DialogControl Control2 Prompt: Plot Map
      mask DialogControl Control2 Callback: MSK_PlotTMap_TMATS()
  Product : Product
  Product1 : Product
  S36 Static Calc : Subsystem
  S36bus : Subsystem
  FlwOut : Outport
  NErr3 : Outport  Port=2
  NErr4 : Outport  Port=3
  HPC_Trq : Outport  Port=4
  HPT_Trq : Outport  Port=5
  C_Data : Outport  Port=6
  wires:
  [S3all] -> Bus Creator/1  "S3"
  [HPC_TrqOut] -> Bus Creator/5  "Trq_HPC"
  [HPS_Nmech] -> Bus Creator/3  "N_HPC"
  Bus Creator/1 -> C_Data/1
  [S4] -> Bus Creator/2  "S4"
  [HPT_TrqOut] -> Bus Creator/6  "Trq_HPT"
  [HPCD] -> Bus Creator/7  "HPC_Data"
  [HPS_Nmech] -> Bus Creator/4  "N_HPT"
  [HPTD] -> Bus Creator/8  "HPT_Data"
  [HPC_Fbld] -> Display/1, HPT/1(CoolingFlwCharIn)
  HPC/5(TrqOut) -> [HPC_TrqOut]
  Burner/1 -> HPT/2(GasPthCharIn), [S4]
  HPC/3(GasPthCharOut) -> Bus Selector1/1, [S3], Burner/2
  [HPT_PRin] -> HPT/3(PRIn)
  HPC/2(FBldsCharOut) -> [HPC_Fbld]
  HPC/1(CustBldsCharOut) -> Compressor_term2/1
  HPT/4(T_Data) -> [HPTD]
  [HPS_Nmech] -> HPT/4(Nmech)
  HPT/3(TrqOut) -> [HPT_TrqOut]
  HPT/2(NErr) -> [HPT_NErr]
  HPT/1(GasPthCharOut) -> [HPTFlowOut]
  [Wf] -> Burner/1, Display5/1
  [HPS_Nmech] -> HPC/3(Nmech)
  Burner/2 -> Burner_term1/1
  [HPC_Rline] -> HPC/2(Rline)
  HPC/4(NErr) -> [HPC_NErr]
  Bus Selector1/1 -> Display7/1  "<W>"
  HPC/6(C_Data) -> [HPCD]
  [HPT_TrqOut] -> HPT_Trq/1
  [HPTFlowOut] -> FlwOut/1
  [HPT_NErr] -> NErr4/1
  [HPC_TrqOut] -> HPC_Trq/1
  [HPC_NErr] -> NErr3/1
  FlwIn/1 -> HPC/1(GasPthCharIn)
  HPS_Nmech/1 -> [HPS_Nmech]
  Wf/1 -> [Wf]
  HPC_Rline/1 -> [HPC_Rline]
  HPT_PRIn/1 -> [HPT_PRin]
  [S3] -> S36 Static Calc/1(S36t)
  S36 Static Calc/1(S36stc) -> [S36stat]
  [S3] -> S36bus/1(S36tot)
  [S36stat] -> S36bus/2(S36stat)
  S36bus/1(S36all) -> [S3all]
  Constant4/1 -> Product/1
  Product/1 -> HPC/4(HP_Mods)
  1/1 -> Product/2
  Time/1 -> [time]
  [time] -> 1/1
  Constant1/1 -> Product1/1
  2/1 -> Product1/2
  [time] -> 2/1
  Product1/1 -> HPT/5(HP_Mods)
